simulink model "Book2222"  (R2019b)
settings: Solver=ode4  StartTime=0.0  StopTime=10.0  FixedStep=0.001  RelTol=1e-3
settings Model: Creator=user  LastModifiedBy=xyh

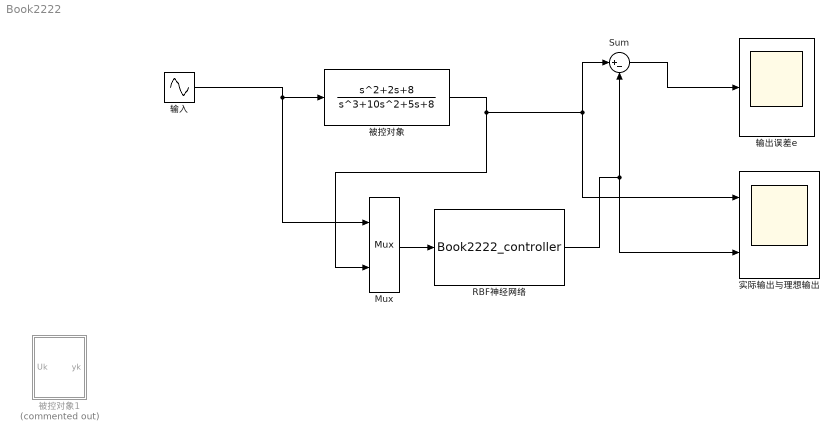
== system Book2222 ==
  Mux : Mux  Inputs=2
  RBF神经网络 : S-Function  FunctionName=Book2222_controller  SFunctionDeploymentMode=off  EnableBusSupport=off
  Sum : Sum  Inputs=|+-
  实际输出与理想输出 : Scope  NumInputPorts=2
  被控对象 : TransferFcn  Numerator=[1 2 8]  Denominator=[1 10 5 8]
  被控对象1 : Subsystem  Commented=on
  输入 : Sin  SampleTime=0
  输出误差e : Scope
  wires:
  被控对象/1 -> Mux/2, Sum/1, 实际输出与理想输出/1
  RBF神经网络/1 -> 实际输出与理想输出/2, Sum/2
  Mux/1 -> RBF神经网络/1
  输入/1 -> Mux/1, 被控对象/1
  Sum/1 -> 输出误差e/1

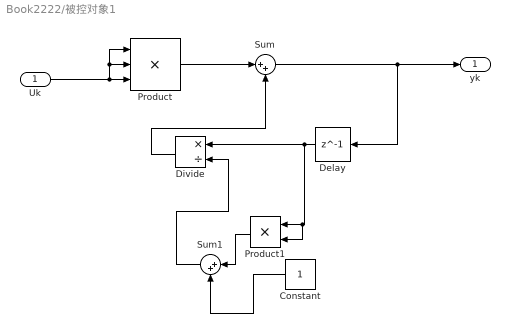
== system Book2222/被控对象1 ==
  Uk : Inport
  Constant : Constant
  Delay : Delay  DelayLength=1
  Divide : Product  Inputs=*/
  Product : Product  Inputs=3
  Product1 : Product
  Sum : Sum  Inputs=|++
  Sum1 : Sum  Inputs=|++
  yk : Outport
  wires:
  Constant/1 -> Sum1/2
  Delay/1 -> Product1/2, Product1/1, Divide/1
  Product/1 -> Sum/1
  Uk/1 -> Product/1, Product/2, Product/3
  Divide/1 -> Sum/2
  Sum/1 -> yk/1, Delay/1
  Product1/1 -> Sum1/1
  Sum1/1 -> Divide/2
